simulink model "Modell_PADDELEC_RB_V3"  (R2019b)
settings: Solver=FixedStepAuto  StartTime=0.0  StopTime=269.98659999999654  FixedStep=0.1  RelTol=1e-3
model workspace (MAT data in the model file):
  SDO_OutputTimes = [0 0.00219999999536 0.0177999999942 0.0334999999977 0.0399999999936 0.0490999999965 0.0497999999934 0.0646999999954 0.0799999999945 0.0802999999942 0.0959000000003 0.111599999997 ... (25110 elements, 25110x1)]
values from neighbouring files (symbols this model uses):
  BAT = clsBattery    [start.m]
  BLDC = clsBLDC    [start.m]
  BoatHull = clsBoatHull    [start.m]
  MotorECU = clsMotorECU    [start.m]
libraries: fl_lib x51, nesl_utility x28, ee_lib x3, simulink x2, eeGeneralControl x1
(part 1 of 2)
settings Model: OrderedModelArguments=off  Creator=Labor-PC  LastModifiedBy=Rene Budich
settings DataIOCC: OutputOption=AdditionalOutputTimes  OutputTimes=SDO_OutputTimes  ReturnWorkspaceOutputsName=SDOSimTest_Log
settings DebuggingCC: ArithmeticOperatorsInVariantConditions=warning
settings SFSimCC: SimUseLocalCustomCode=off  CustomCodeUndefinedFunction=UseInterfaceOnly
settings RTWCC: RTWUseLocalCustomCode=off

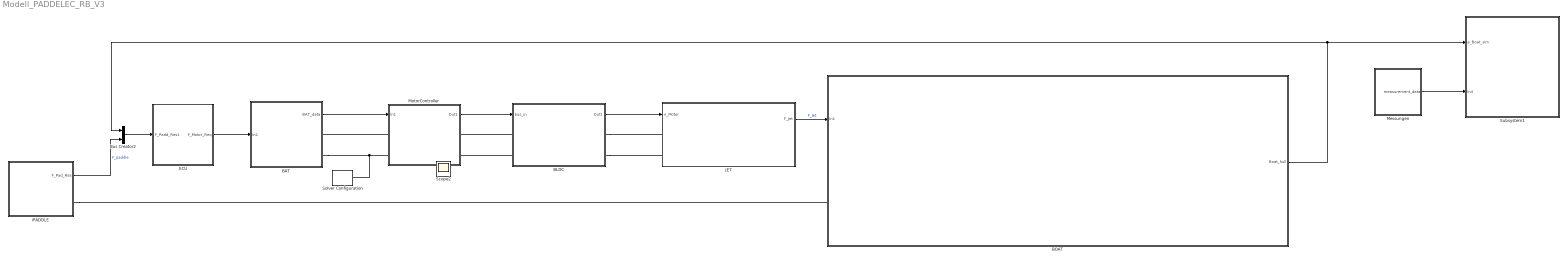
== system Modell_PADDELEC_RB_V3 ==
  BAT : Subsystem
      mask Display: image('Battery.jpg'); % Use "Edit Image" on toolstrip to change.
  BLDC : Subsystem
      mask Display: image('Motor.png'); % Use "Edit Image" on toolstrip to change.
  BOAT : Subsystem
      mask Display: image('D:\00_Sandbox\Matlab\Modell_20200324\03_symbols\Kajak.png'); % Use "Edit Image" on toolstrip to change.
  Bus Creator2 : BusCreator  Inputs=2
  ECU : Subsystem
      mask Display: image('D:\00_Sandbox\Matlab\Modell_20200324\03_symbols\ECU.png'); % Use "Edit Image" on toolstrip to change.
  "JET " : Subsystem
      mask Display: image('D:\00_Sandbox\Matlab\Modell_20200324\03_symbols\Jet.PNG'); % Use "Edit Image" on toolstrip to change.
  Messungen : Subsystem
      mask Display: image('D:\00_Sandbox\Matlab\Modell_20200324\03_symbols\Measurement.png'); % Use "Edit Image" on toolstrip to change.
  MotorController : Subsystem
      mask Display: image('MotorECU.jpg'); % Use "Edit Image" on toolstrip to change.
  Solver Configuration : nesl_utility/Solver Configuration  PhysicalDomain=network_engine_domain  SubClassName=solver  LeftPortType=input  RightPortType=generic  Tones=[]  Harmonics=[]  SimulateNoise=off  Profile=off  UseLocalSampling=off  EnableSwitchedLinearOptims=on  FrequencyDomain=off  UseCCode=off  RelTol=0.001  AbsTol=1e-06  MinStep=1e-09  ToWorkspace=off  RevertToSquareIcSolve=off  NumHomotopyIterations=100  PhasorMode=off  PhasorModeNumHarmonics=1  DoDC=off  ResidualTolerance=1e-09  UseLocalSolver=off  LocalSolverChoice=NE_BACKWARD_EULER_ADVANCER  LocalSolverSampleTime=0.001  DoFixedCost=off  MaxNonlinIter=3  MaxModeIter=2  LinearAlgebra=Sparse  EquationFormulation=NE_TIME_EF  DelaysMemoryBudget=1024  AutomaticFiltering=on  FilteringTimeConstant=0.001  PartitionStorageMethod=AS_NEEDED  PartitionMemoryBudget=1024  PartitionMethod=FAST
  Subsystem1 : Subsystem
      mask Display: image('D:\00_Sandbox\Matlab\Modell_20200324\03_symbols\Auswertung.png'); % Use "Edit Image" on toolstrip to change.
  iPADDLE : Subsystem
      mask Display: image('D:\00_Sandbox\Matlab\Modell_20200324\03_symbols\paddle.png'); % Use "Edit Image" on toolstrip to change.
  Scope2 : Scope
  wires:
  Messungen/1(measurement_data) -> Subsystem1/2(In4)
  BOAT/1(Boat_hull) -> Bus Creator2/1, Subsystem1/1(a_Boat_sim)
  MotorController/1(Out1) -> BLDC/1(bus_in)
  "JET "/1(F_Jet) -> BOAT/1(In1)  "F_Jet"
  iPADDLE/1(F_Pad_Res) -> Bus Creator2/2  "F_paddle"
  Bus Creator2/1 -> ECU/1(F_Padd_Res1)
  ECU/1(F_Motor_Req) -> BAT/1(In1)
  BAT/1(BAT_data) -> MotorController/1(In1)
  BLDC/1(Out1) -> "JET "/1(n_Motor)
  connections:
  BLDC/RConn1 -- "JET "/LConn1
  iPADDLE/RConn1 -- BOAT/LConn1
  BAT/RConn2 -- Solver Configuration/RConn1 -- MotorController/LConn2
  BLDC/RConn2 -- "JET "/LConn2
  MotorController/LConn1 -- BAT/RConn1
  BLDC/LConn1 -- MotorController/RConn1
  BLDC/LConn2 -- MotorController/RConn2
